simulink model "RoverA1Arch"  (R2026a)
settings: Solver=VariableStepAuto
model workspace (MAT data in the model file):
  averageLoad = Simulink.Parameter
  averageLoad.Value = 160
  averageLoad.Complexity = 'real'
  averageLoad.Dimensions = [1 1]
  averageLoad.DataType = 'double'
  averageLoad.DocUnits = 'W'
  bodyMass = Simulink.Parameter
  bodyMass.Value = 33.45
  bodyMass.Complexity = 'real'
  bodyMass.Dimensions = [1 1]
  bodyMass.DataType = 'double'
  bodyMass.DocUnits = 'kg'
  wheelSeparation = Simulink.Parameter
  wheelSeparation.Value = 0.62602
  wheelSeparation.Complexity = 'real'
  wheelSeparation.Dimensions = [1 1]
  wheelSeparation.DataType = 'double'
  wheelSeparation.DocUnits = 'm'
  wheelbase = Simulink.Parameter
  wheelbase.Value = 0.5084
  wheelbase.Complexity = 'real'
  wheelbase.Dimensions = [1 1]
  wheelbase.DataType = 'double'
  wheelbase.DocUnits = 'm'
settings Model: DataDictionary=RoverA1Interfaces.sldd  ParameterArgumentNames=bodyMass,wheelSeparation,wheelbase,averageLoad  Creator=potlo  LastModifiedBy=potlo

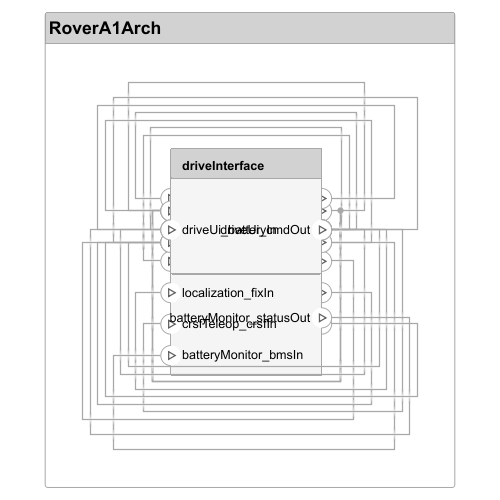
[thumbnail: Simulink's stored preview of the top-level diagram]
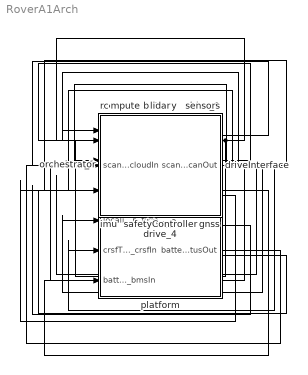
== system RoverA1Arch ==
  battery : Subsystem  mask{capacity=40, nominalVoltage=24}
      settings: PortSchema="{\"entries\":[{\"content\":{\"headerSize\":26,\"margin\":15,\"minimumSpacing\":25,\"sides\":[{\"content\":{},\"type\":\"ConnectorPlacement.EquallySpacedRectSide\",\"uuid\":\"200c6e72-70f4-4dab-9973-1633f40310af\"},{\"content\":{\"connectorIds\":[\"Out1\",\"Out2\"],\"side\":\"RIGHT\"},\"type\":\"ConnectorPlacement.EquallySpacedRectSide\",\"uuid\":\"bbe755dc-37e6-4ccf-babc-f69c624e3127\"},{\"content\":{\"side\":\"TOP\"},\"type\":\"ConnectorPlacement.EquallySpacedRectSide\",\"uuid\":\"af29013d-bc34-4ea7-a3b1-8488eaa61b9f\"}]},\"type\":\"ConnectorPlacement.EquallySpacedConnector\",\"uuid\":\"0c1b5d18-eb5c-4f03-ad77-d46c7555bc12\"}],\"packageUris\":[\"http://schema.mathworks.com/mf0/Connector/R2020b\"],\"version\":\"1.0\"}"
  compute : Subsystem
      settings: PortSchema="{\"entries\":[{\"content\":{\"headerSize\":26,\"margin\":15,\"minimumSpacing\":25,\"sides\":[{\"content\":{},\"type\":\"ConnectorPlacement.EquallySpacedRectSide\",\"uuid\":\"200c6e72-70f4-4dab-9973-1633f40310af\"},{\"content\":{\"connectorIds\":[\"Out1\",\"Out2\",\"Out3\",\"Out4\",\"Out5\"],\"side\":\"RIGHT\"},\"type\":\"ConnectorPlacement.EquallySpacedRectSide\",\"uuid\":\"bbe755dc-37e6-4ccf-babc-f69c624e3127\"},{\"content\":{\"side\":\"TOP\"},\"type\":\"ConnectorPlacement.EquallySpacedRectSide\",\"uuid\":\"af29013d-bc34-4ea7-a3b1-8488eaa61b9f\"}]},\"type\":\"ConnectorPlacement.EquallySpacedConnector\",\"uuid\":\"0c1b5d18-eb5c-4f03-ad77-d46c7555bc12\"}],\"packageUris\":[\"http://schema.mathworks.com/mf0/Connector/R2020b\"],\"version\":\"1.0\"}"
  driveInterface : Subsystem
      settings: PortSchema="{\"entries\":[{\"content\":{\"headerSize\":26,\"margin\":15,\"minimumSpacing\":25,\"sides\":[{\"content\":{\"connectorIds\":[\"In1\"]},\"type\":\"ConnectorPlacement.EquallySpacedRectSide\",\"uuid\":\"200c6e72-70f4-4dab-9973-1633f40310af\"},{\"content\":{\"connectorIds\":[\"Out1\"],\"side\":\"RIGHT\"},\"type\":\"ConnectorPlacement.EquallySpacedRectSide\",\"uuid\":\"bbe755dc-37e6-4ccf-babc-f69c624e3127\"},{\"content\":{\"side\":\"TOP\"},\"type\":\"ConnectorPlacement.EquallySpacedRectSide\",\"uuid\":\"af29013d-bc34-4ea7-a3b1-8488eaa61b9f\"}]},\"type\":\"ConnectorPlacement.EquallySpacedConnector\",\"uuid\":\"0c1b5d18-eb5c-4f03-ad77-d46c7555bc12\"}],\"packageUris\":[\"http://schema.mathworks.com/mf0/Connector/R2020b\"],\"version\":\"1.0\"}"
  drive_1 : Subsystem
      settings: PortSchema="{\"entries\":[{\"content\":{\"headerSize\":26,\"margin\":15,\"minimumSpacing\":25,\"sides\":[{\"content\":{\"connectorIds\":[\"In1\",\"In2\"]},\"type\":\"ConnectorPlacement.EquallySpacedRectSide\",\"uuid\":\"200c6e72-70f4-4dab-9973-1633f40310af\"},{\"content\":{\"side\":\"RIGHT\"},\"type\":\"ConnectorPlacement.EquallySpacedRectSide\",\"uuid\":\"bbe755dc-37e6-4ccf-babc-f69c624e3127\"},{\"content\":{\"side\":\"TOP\"},\"type\":\"ConnectorPlacement.EquallySpacedRectSide\",\"uuid\":\"af29013d-bc34-4ea7-a3b1-8488eaa61b9f\"}]},\"type\":\"ConnectorPlacement.EquallySpacedConnector\",\"uuid\":\"0c1b5d18-eb5c-4f03-ad77-d46c7555bc12\"}],\"packageUris\":[\"http://schema.mathworks.com/mf0/Connector/R2020b\"],\"version\":\"1.0\"}"
  drive_2 : Subsystem
      settings: PortSchema="{\"entries\":[{\"content\":{\"headerSize\":26,\"margin\":15,\"minimumSpacing\":25,\"sides\":[{\"content\":{\"connectorIds\":[\"In1\",\"In2\"]},\"type\":\"ConnectorPlacement.EquallySpacedRectSide\",\"uuid\":\"200c6e72-70f4-4dab-9973-1633f40310af\"},{\"content\":{\"side\":\"RIGHT\"},\"type\":\"ConnectorPlacement.EquallySpacedRectSide\",\"uuid\":\"bbe755dc-37e6-4ccf-babc-f69c624e3127\"},{\"content\":{\"side\":\"TOP\"},\"type\":\"ConnectorPlacement.EquallySpacedRectSide\",\"uuid\":\"af29013d-bc34-4ea7-a3b1-8488eaa61b9f\"}]},\"type\":\"ConnectorPlacement.EquallySpacedConnector\",\"uuid\":\"0c1b5d18-eb5c-4f03-ad77-d46c7555bc12\"}],\"packageUris\":[\"http://schema.mathworks.com/mf0/Connector/R2020b\"],\"version\":\"1.0\"}"
  drive_3 : Subsystem
      settings: PortSchema="{\"entries\":[{\"content\":{\"headerSize\":26,\"margin\":15,\"minimumSpacing\":25,\"sides\":[{\"content\":{\"connectorIds\":[\"In1\",\"In2\"]},\"type\":\"ConnectorPlacement.EquallySpacedRectSide\",\"uuid\":\"200c6e72-70f4-4dab-9973-1633f40310af\"},{\"content\":{\"side\":\"RIGHT\"},\"type\":\"ConnectorPlacement.EquallySpacedRectSide\",\"uuid\":\"bbe755dc-37e6-4ccf-babc-f69c624e3127\"},{\"content\":{\"side\":\"TOP\"},\"type\":\"ConnectorPlacement.EquallySpacedRectSide\",\"uuid\":\"af29013d-bc34-4ea7-a3b1-8488eaa61b9f\"}]},\"type\":\"ConnectorPlacement.EquallySpacedConnector\",\"uuid\":\"0c1b5d18-eb5c-4f03-ad77-d46c7555bc12\"}],\"packageUris\":[\"http://schema.mathworks.com/mf0/Connector/R2020b\"],\"version\":\"1.0\"}"
  drive_4 : Subsystem
      settings: PortSchema="{\"entries\":[{\"content\":{\"headerSize\":26,\"margin\":15,\"minimumSpacing\":25,\"sides\":[{\"content\":{\"connectorIds\":[\"In1\",\"In2\"]},\"type\":\"ConnectorPlacement.EquallySpacedRectSide\",\"uuid\":\"200c6e72-70f4-4dab-9973-1633f40310af\"},{\"content\":{\"side\":\"RIGHT\"},\"type\":\"ConnectorPlacement.EquallySpacedRectSide\",\"uuid\":\"bbe755dc-37e6-4ccf-babc-f69c624e3127\"},{\"content\":{\"side\":\"TOP\"},\"type\":\"ConnectorPlacement.EquallySpacedRectSide\",\"uuid\":\"af29013d-bc34-4ea7-a3b1-8488eaa61b9f\"}]},\"type\":\"ConnectorPlacement.EquallySpacedConnector\",\"uuid\":\"0c1b5d18-eb5c-4f03-ad77-d46c7555bc12\"}],\"packageUris\":[\"http://schema.mathworks.com/mf0/Connector/R2020b\"],\"version\":\"1.0\"}"
  gnss : Subsystem  mask{fixRate=1}
      settings: PortSchema="{\"entries\":[{\"content\":{\"headerSize\":26,\"margin\":15,\"minimumSpacing\":25,\"sides\":[{\"content\":{},\"type\":\"ConnectorPlacement.EquallySpacedRectSide\",\"uuid\":\"200c6e72-70f4-4dab-9973-1633f40310af\"},{\"content\":{\"connectorIds\":[\"Out1\"],\"side\":\"RIGHT\"},\"type\":\"ConnectorPlacement.EquallySpacedRectSide\",\"uuid\":\"bbe755dc-37e6-4ccf-babc-f69c624e3127\"},{\"content\":{\"side\":\"TOP\"},\"type\":\"ConnectorPlacement.EquallySpacedRectSide\",\"uuid\":\"af29013d-bc34-4ea7-a3b1-8488eaa61b9f\"}]},\"type\":\"ConnectorPlacement.EquallySpacedConnector\",\"uuid\":\"0c1b5d18-eb5c-4f03-ad77-d46c7555bc12\"}],\"packageUris\":[\"http://schema.mathworks.com/mf0/Connector/R2020b\"],\"version\":\"1.0\"}"
  imu : Subsystem
      settings: PortSchema="{\"entries\":[{\"content\":{\"headerSize\":26,\"margin\":15,\"minimumSpacing\":25,\"sides\":[{\"content\":{},\"type\":\"ConnectorPlacement.EquallySpacedRectSide\",\"uuid\":\"200c6e72-70f4-4dab-9973-1633f40310af\"},{\"content\":{\"connectorIds\":[\"Out1\"],\"side\":\"RIGHT\"},\"type\":\"ConnectorPlacement.EquallySpacedRectSide\",\"uuid\":\"bbe755dc-37e6-4ccf-babc-f69c624e3127\"},{\"content\":{\"side\":\"TOP\"},\"type\":\"ConnectorPlacement.EquallySpacedRectSide\",\"uuid\":\"af29013d-bc34-4ea7-a3b1-8488eaa61b9f\"}]},\"type\":\"ConnectorPlacement.EquallySpacedConnector\",\"uuid\":\"0c1b5d18-eb5c-4f03-ad77-d46c7555bc12\"}],\"packageUris\":[\"http://schema.mathworks.com/mf0/Connector/R2020b\"],\"version\":\"1.0\"}"
  lidar : Subsystem  mask{scanRate=10}
      settings: PortSchema="{\"entries\":[{\"content\":{\"headerSize\":26,\"margin\":15,\"minimumSpacing\":25,\"sides\":[{\"content\":{},\"type\":\"ConnectorPlacement.EquallySpacedRectSide\",\"uuid\":\"200c6e72-70f4-4dab-9973-1633f40310af\"},{\"content\":{\"connectorIds\":[\"Out1\"],\"side\":\"RIGHT\"},\"type\":\"ConnectorPlacement.EquallySpacedRectSide\",\"uuid\":\"bbe755dc-37e6-4ccf-babc-f69c624e3127\"},{\"content\":{\"side\":\"TOP\"},\"type\":\"ConnectorPlacement.EquallySpacedRectSide\",\"uuid\":\"af29013d-bc34-4ea7-a3b1-8488eaa61b9f\"}]},\"type\":\"ConnectorPlacement.EquallySpacedConnector\",\"uuid\":\"0c1b5d18-eb5c-4f03-ad77-d46c7555bc12\"}],\"packageUris\":[\"http://schema.mathworks.com/mf0/Connector/R2020b\"],\"version\":\"1.0\"}"
  orchestrator : Subsystem
      settings: PortSchema="{\"entries\":[{\"content\":{\"headerSize\":26,\"margin\":15,\"minimumSpacing\":25,\"sides\":[{\"content\":{\"connectorIds\":[\"In1\",\"In2\"]},\"type\":\"ConnectorPlacement.EquallySpacedRectSide\",\"uuid\":\"200c6e72-70f4-4dab-9973-1633f40310af\"},{\"content\":{\"connectorIds\":[\"Out1\"],\"side\":\"RIGHT\"},\"type\":\"ConnectorPlacement.EquallySpacedRectSide\",\"uuid\":\"bbe755dc-37e6-4ccf-babc-f69c624e3127\"},{\"content\":{\"side\":\"TOP\"},\"type\":\"ConnectorPlacement.EquallySpacedRectSide\",\"uuid\":\"af29013d-bc34-4ea7-a3b1-8488eaa61b9f\"}]},\"type\":\"ConnectorPlacement.EquallySpacedConnector\",\"uuid\":\"0c1b5d18-eb5c-4f03-ad77-d46c7555bc12\"}],\"packageUris\":[\"http://schema.mathworks.com/mf0/Connector/R2020b\"],\"version\":\"1.0\"}"
  platform : Subsystem
      settings: PortSchema="{\"entries\":[{\"content\":{\"headerSize\":26,\"margin\":15,\"minimumSpacing\":25,\"sides\":[{\"content\":{\"connectorIds\":[\"In1\",\"In2\",\"In3\",\"In4\",\"In5\",\"In6\"]},\"type\":\"ConnectorPlacement.EquallySpacedRectSide\",\"uuid\":\"200c6e72-70f4-4dab-9973-1633f40310af\"},{\"content\":{\"connectorIds\":[\"Out1\",\"Out2\"],\"side\":\"RIGHT\"},\"type\":\"ConnectorPlacement.EquallySpacedRectSide\",\"uuid\":\"bbe755dc-37e6-4ccf-babc-f69c624e3127\"},{\"content\":{\"side\":\"TOP\"},\"type\":\"ConnectorPlacement.EquallySpacedRectSide\",\"uuid\":\"af29013d-bc34-4ea7-a3b1-8488eaa61b9f\"}]},\"type\":\"ConnectorPlacement.EquallySpacedConnector\",\"uuid\":\"0c1b5d18-eb5c-4f03-ad77-d46c7555bc12\"}],\"packageUris\":[\"http://schema.mathworks.com/mf0/Connector/R2020b\"],\"version\":\"1.0\"}"
  rc : Subsystem
      settings: PortSchema="{\"entries\":[{\"content\":{\"headerSize\":26,\"margin\":15,\"minimumSpacing\":25,\"sides\":[{\"content\":{},\"type\":\"ConnectorPlacement.EquallySpacedRectSide\",\"uuid\":\"200c6e72-70f4-4dab-9973-1633f40310af\"},{\"content\":{\"connectorIds\":[\"Out1\"],\"side\":\"RIGHT\"},\"type\":\"ConnectorPlacement.EquallySpacedRectSide\",\"uuid\":\"bbe755dc-37e6-4ccf-babc-f69c624e3127\"},{\"content\":{\"side\":\"TOP\"},\"type\":\"ConnectorPlacement.EquallySpacedRectSide\",\"uuid\":\"af29013d-bc34-4ea7-a3b1-8488eaa61b9f\"}]},\"type\":\"ConnectorPlacement.EquallySpacedConnector\",\"uuid\":\"0c1b5d18-eb5c-4f03-ad77-d46c7555bc12\"}],\"packageUris\":[\"http://schema.mathworks.com/mf0/Connector/R2020b\"],\"version\":\"1.0\"}"
  safetyController : Subsystem  mask{watchdogPeriod=0.2}
      settings: PortSchema="{\"entries\":[{\"content\":{\"headerSize\":26,\"margin\":15,\"minimumSpacing\":25,\"sides\":[{\"content\":{\"connectorIds\":[\"In1\"]},\"type\":\"ConnectorPlacement.EquallySpacedRectSide\",\"uuid\":\"200c6e72-70f4-4dab-9973-1633f40310af\"},{\"content\":{\"side\":\"RIGHT\"},\"type\":\"ConnectorPlacement.EquallySpacedRectSide\",\"uuid\":\"bbe755dc-37e6-4ccf-babc-f69c624e3127\"},{\"content\":{\"side\":\"TOP\"},\"type\":\"ConnectorPlacement.EquallySpacedRectSide\",\"uuid\":\"af29013d-bc34-4ea7-a3b1-8488eaa61b9f\"}]},\"type\":\"ConnectorPlacement.EquallySpacedConnector\",\"uuid\":\"0c1b5d18-eb5c-4f03-ad77-d46c7555bc12\"}],\"packageUris\":[\"http://schema.mathworks.com/mf0/Connector/R2020b\"],\"version\":\"1.0\"}"
  sensors : Subsystem
      settings: PortSchema="{\"entries\":[{\"content\":{\"headerSize\":26,\"margin\":15,\"minimumSpacing\":25,\"sides\":[{\"content\":{\"connectorIds\":[\"In1\"]},\"type\":\"ConnectorPlacement.EquallySpacedRectSide\",\"uuid\":\"200c6e72-70f4-4dab-9973-1633f40310af\"},{\"content\":{\"connectorIds\":[\"Out1\"],\"side\":\"RIGHT\"},\"type\":\"ConnectorPlacement.EquallySpacedRectSide\",\"uuid\":\"bbe755dc-37e6-4ccf-babc-f69c624e3127\"},{\"content\":{\"side\":\"TOP\"},\"type\":\"ConnectorPlacement.EquallySpacedRectSide\",\"uuid\":\"af29013d-bc34-4ea7-a3b1-8488eaa61b9f\"}]},\"type\":\"ConnectorPlacement.EquallySpacedConnector\",\"uuid\":\"0c1b5d18-eb5c-4f03-ad77-d46c7555bc12\"}],\"packageUris\":[\"http://schema.mathworks.com/mf0/Connector/R2020b\"],\"version\":\"1.0\"}"
  wires:
  driveInterface/1(driveUi_cmdOut) -> platform/1(twistMux_webIn)
  orchestrator/1(navigation_cmdOut) -> platform/2(twistMux_navIn)
  imu/1(imuOut) -> platform/3(localization_imuIn)
  gnss/1(fixOut) -> platform/4(localization_fixIn)
  platform/1(localization_odomOut) -> orchestrator/1(navigation_odomIn)
  lidar/1(cloudOut) -> sensors/1(scanProjection_cloudIn)
  sensors/1(scanProjection_scanOut) -> orchestrator/2(navigation_scanIn)
  battery/1(powerOut) -> drive_1/1(controller_powerIn), drive_2/1(controller_powerIn), drive_3/1(controller_powerIn), drive_4/1(controller_powerIn)
  compute/2(wheelCmdOut_1) -> drive_1/2(controller_wheelCmdIn)
  compute/3(wheelCmdOut_2) -> drive_2/2(controller_wheelCmdIn)
  compute/4(wheelCmdOut_3) -> drive_3/2(controller_wheelCmdIn)
  compute/5(wheelCmdOut_4) -> drive_4/2(controller_wheelCmdIn)
  rc/1(crsfOut) -> platform/5(crsfTeleop_crsfIn)
  battery/2(statusOut) -> platform/6(batteryMonitor_bmsIn)
  platform/2(batteryMonitor_statusOut) -> driveInterface/1(driveUi_batteryIn)
  compute/1(modbus) -> safetyController/1(modbus)

== system RoverA1Arch/battery ==
  Bus Element Out1 : Outport  PortName=powerOut
  Bus Element Out2 : Outport  Port=2  PortName=statusOut

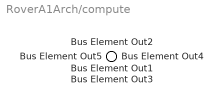
== system RoverA1Arch/compute ==
  Bus Element Out1 : Outport  PortName=modbus
  Bus Element Out2 : Outport  Port=2  PortName=wheelCmdOut_1
  Bus Element Out3 : Outport  Port=3  PortName=wheelCmdOut_2
  Bus Element Out4 : Outport  Port=4  PortName=wheelCmdOut_3
  Bus Element Out5 : Outport  Port=5  PortName=wheelCmdOut_4

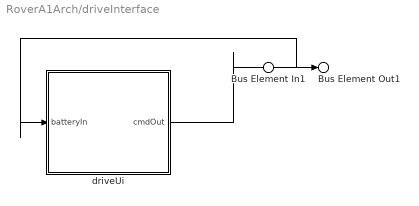
== system RoverA1Arch/driveInterface ==
  Bus Element In1 : Inport  PortName=driveUi_batteryIn
  driveUi : Subsystem
      settings: PortSchema="{\"entries\":[{\"content\":{\"headerSize\":26,\"margin\":15,\"minimumSpacing\":25,\"sides\":[{\"content\":{\"connectorIds\":[\"In1\"]},\"type\":\"ConnectorPlacement.EquallySpacedRectSide\",\"uuid\":\"200c6e72-70f4-4dab-9973-1633f40310af\"},{\"content\":{\"connectorIds\":[\"Out1\"],\"side\":\"RIGHT\"},\"type\":\"ConnectorPlacement.EquallySpacedRectSide\",\"uuid\":\"bbe755dc-37e6-4ccf-babc-f69c624e3127\"},{\"content\":{\"side\":\"TOP\"},\"type\":\"ConnectorPlacement.EquallySpacedRectSide\",\"uuid\":\"af29013d-bc34-4ea7-a3b1-8488eaa61b9f\"}]},\"type\":\"ConnectorPlacement.EquallySpacedConnector\",\"uuid\":\"0c1b5d18-eb5c-4f03-ad77-d46c7555bc12\"}],\"packageUris\":[\"http://schema.mathworks.com/mf0/Connector/R2020b\"],\"version\":\"1.0\"}"
  Bus Element Out1 : Outport  PortName=driveUi_cmdOut
  wires:
  driveUi/1(cmdOut) -> Bus Element Out1/1
  Bus Element In1/1 -> driveUi/1(batteryIn)

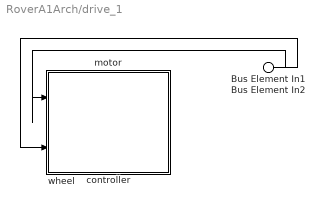
== system RoverA1Arch/drive_1 ==
  Bus Element In1 : Inport  PortName=controller_powerIn
  Bus Element In2 : Inport  Port=2  PortName=controller_wheelCmdIn
  controller : Subsystem
      settings: PortSchema="{\"entries\":[{\"content\":{\"headerSize\":26,\"margin\":15,\"minimumSpacing\":25,\"sides\":[{\"content\":{\"connectorIds\":[\"In1\",\"In2\"]},\"type\":\"ConnectorPlacement.EquallySpacedRectSide\",\"uuid\":\"200c6e72-70f4-4dab-9973-1633f40310af\"},{\"content\":{\"side\":\"RIGHT\"},\"type\":\"ConnectorPlacement.EquallySpacedRectSide\",\"uuid\":\"bbe755dc-37e6-4ccf-babc-f69c624e3127\"},{\"content\":{\"side\":\"TOP\"},\"type\":\"ConnectorPlacement.EquallySpacedRectSide\",\"uuid\":\"af29013d-bc34-4ea7-a3b1-8488eaa61b9f\"}]},\"type\":\"ConnectorPlacement.EquallySpacedConnector\",\"uuid\":\"0c1b5d18-eb5c-4f03-ad77-d46c7555bc12\"}],\"packageUris\":[\"http://schema.mathworks.com/mf0/Connector/R2020b\"],\"version\":\"1.0\"}"
  motor : Subsystem  mask{noLoadSpeed=293.2, gearRatio=23.3, gearboxEfficiency=0.70, currentLimit=15, jointVelocityLimit=10.958}
      settings: PortSchema="{\"entries\":[{\"content\":{\"headerSize\":26,\"margin\":15,\"minimumSpacing\":25,\"sides\":[{\"content\":{},\"type\":\"ConnectorPlacement.EquallySpacedRectSide\",\"uuid\":\"200c6e72-70f4-4dab-9973-1633f40310af\"},{\"content\":{\"side\":\"RIGHT\"},\"type\":\"ConnectorPlacement.EquallySpacedRectSide\",\"uuid\":\"bbe755dc-37e6-4ccf-babc-f69c624e3127\"},{\"content\":{\"side\":\"TOP\"},\"type\":\"ConnectorPlacement.EquallySpacedRectSide\",\"uuid\":\"af29013d-bc34-4ea7-a3b1-8488eaa61b9f\"}]},\"type\":\"ConnectorPlacement.EquallySpacedConnector\",\"uuid\":\"0c1b5d18-eb5c-4f03-ad77-d46c7555bc12\"}],\"packageUris\":[\"http://schema.mathworks.com/mf0/Connector/R2020b\"],\"version\":\"1.0\"}"
  wheel : Subsystem  mask{radius=0.1651, width=0.108, mass=2.5}
      settings: PortSchema="{\"entries\":[{\"content\":{\"headerSize\":26,\"margin\":15,\"minimumSpacing\":25,\"sides\":[{\"content\":{},\"type\":\"ConnectorPlacement.EquallySpacedRectSide\",\"uuid\":\"200c6e72-70f4-4dab-9973-1633f40310af\"},{\"content\":{\"side\":\"RIGHT\"},\"type\":\"ConnectorPlacement.EquallySpacedRectSide\",\"uuid\":\"bbe755dc-37e6-4ccf-babc-f69c624e3127\"},{\"content\":{\"side\":\"TOP\"},\"type\":\"ConnectorPlacement.EquallySpacedRectSide\",\"uuid\":\"af29013d-bc34-4ea7-a3b1-8488eaa61b9f\"}]},\"type\":\"ConnectorPlacement.EquallySpacedConnector\",\"uuid\":\"0c1b5d18-eb5c-4f03-ad77-d46c7555bc12\"}],\"packageUris\":[\"http://schema.mathworks.com/mf0/Connector/R2020b\"],\"version\":\"1.0\"}"
  wires:
  Bus Element In1/1 -> controller/2(powerIn)
  Bus Element In2/1 -> controller/1(wheelCmdIn)

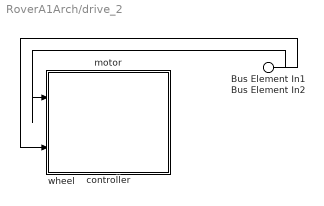
== system RoverA1Arch/drive_2 ==
  Bus Element In1 : Inport  PortName=controller_powerIn
  Bus Element In2 : Inport  Port=2  PortName=controller_wheelCmdIn
  controller : Subsystem
      settings: PortSchema="{\"entries\":[{\"content\":{\"headerSize\":26,\"margin\":15,\"minimumSpacing\":25,\"sides\":[{\"content\":{\"connectorIds\":[\"In1\",\"In2\"]},\"type\":\"ConnectorPlacement.EquallySpacedRectSide\",\"uuid\":\"200c6e72-70f4-4dab-9973-1633f40310af\"},{\"content\":{\"side\":\"RIGHT\"},\"type\":\"ConnectorPlacement.EquallySpacedRectSide\",\"uuid\":\"bbe755dc-37e6-4ccf-babc-f69c624e3127\"},{\"content\":{\"side\":\"TOP\"},\"type\":\"ConnectorPlacement.EquallySpacedRectSide\",\"uuid\":\"af29013d-bc34-4ea7-a3b1-8488eaa61b9f\"}]},\"type\":\"ConnectorPlacement.EquallySpacedConnector\",\"uuid\":\"0c1b5d18-eb5c-4f03-ad77-d46c7555bc12\"}],\"packageUris\":[\"http://schema.mathworks.com/mf0/Connector/R2020b\"],\"version\":\"1.0\"}"
  motor : Subsystem  mask{noLoadSpeed=293.2, gearRatio=23.3, gearboxEfficiency=0.70, currentLimit=15, jointVelocityLimit=10.958}
      settings: PortSchema="{\"entries\":[{\"content\":{\"headerSize\":26,\"margin\":15,\"minimumSpacing\":25,\"sides\":[{\"content\":{},\"type\":\"ConnectorPlacement.EquallySpacedRectSide\",\"uuid\":\"200c6e72-70f4-4dab-9973-1633f40310af\"},{\"content\":{\"side\":\"RIGHT\"},\"type\":\"ConnectorPlacement.EquallySpacedRectSide\",\"uuid\":\"bbe755dc-37e6-4ccf-babc-f69c624e3127\"},{\"content\":{\"side\":\"TOP\"},\"type\":\"ConnectorPlacement.EquallySpacedRectSide\",\"uuid\":\"af29013d-bc34-4ea7-a3b1-8488eaa61b9f\"}]},\"type\":\"ConnectorPlacement.EquallySpacedConnector\",\"uuid\":\"0c1b5d18-eb5c-4f03-ad77-d46c7555bc12\"}],\"packageUris\":[\"http://schema.mathworks.com/mf0/Connector/R2020b\"],\"version\":\"1.0\"}"
  wheel : Subsystem  mask{radius=0.1651, width=0.108, mass=2.5}
      settings: PortSchema="{\"entries\":[{\"content\":{\"headerSize\":26,\"margin\":15,\"minimumSpacing\":25,\"sides\":[{\"content\":{},\"type\":\"ConnectorPlacement.EquallySpacedRectSide\",\"uuid\":\"200c6e72-70f4-4dab-9973-1633f40310af\"},{\"content\":{\"side\":\"RIGHT\"},\"type\":\"ConnectorPlacement.EquallySpacedRectSide\",\"uuid\":\"bbe755dc-37e6-4ccf-babc-f69c624e3127\"},{\"content\":{\"side\":\"TOP\"},\"type\":\"ConnectorPlacement.EquallySpacedRectSide\",\"uuid\":\"af29013d-bc34-4ea7-a3b1-8488eaa61b9f\"}]},\"type\":\"ConnectorPlacement.EquallySpacedConnector\",\"uuid\":\"0c1b5d18-eb5c-4f03-ad77-d46c7555bc12\"}],\"packageUris\":[\"http://schema.mathworks.com/mf0/Connector/R2020b\"],\"version\":\"1.0\"}"
  wires:
  Bus Element In1/1 -> controller/2(powerIn)
  Bus Element In2/1 -> controller/1(wheelCmdIn)

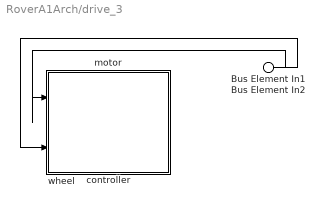
== system RoverA1Arch/drive_3 ==
  Bus Element In1 : Inport  PortName=controller_powerIn
  Bus Element In2 : Inport  Port=2  PortName=controller_wheelCmdIn
  controller : Subsystem
      settings: PortSchema="{\"entries\":[{\"content\":{\"headerSize\":26,\"margin\":15,\"minimumSpacing\":25,\"sides\":[{\"content\":{\"connectorIds\":[\"In1\",\"In2\"]},\"type\":\"ConnectorPlacement.EquallySpacedRectSide\",\"uuid\":\"200c6e72-70f4-4dab-9973-1633f40310af\"},{\"content\":{\"side\":\"RIGHT\"},\"type\":\"ConnectorPlacement.EquallySpacedRectSide\",\"uuid\":\"bbe755dc-37e6-4ccf-babc-f69c624e3127\"},{\"content\":{\"side\":\"TOP\"},\"type\":\"ConnectorPlacement.EquallySpacedRectSide\",\"uuid\":\"af29013d-bc34-4ea7-a3b1-8488eaa61b9f\"}]},\"type\":\"ConnectorPlacement.EquallySpacedConnector\",\"uuid\":\"0c1b5d18-eb5c-4f03-ad77-d46c7555bc12\"}],\"packageUris\":[\"http://schema.mathworks.com/mf0/Connector/R2020b\"],\"version\":\"1.0\"}"
  motor : Subsystem  mask{noLoadSpeed=293.2, gearRatio=23.3, gearboxEfficiency=0.70, currentLimit=15, jointVelocityLimit=10.958}
      settings: PortSchema="{\"entries\":[{\"content\":{\"headerSize\":26,\"margin\":15,\"minimumSpacing\":25,\"sides\":[{\"content\":{},\"type\":\"ConnectorPlacement.EquallySpacedRectSide\",\"uuid\":\"200c6e72-70f4-4dab-9973-1633f40310af\"},{\"content\":{\"side\":\"RIGHT\"},\"type\":\"ConnectorPlacement.EquallySpacedRectSide\",\"uuid\":\"bbe755dc-37e6-4ccf-babc-f69c624e3127\"},{\"content\":{\"side\":\"TOP\"},\"type\":\"ConnectorPlacement.EquallySpacedRectSide\",\"uuid\":\"af29013d-bc34-4ea7-a3b1-8488eaa61b9f\"}]},\"type\":\"ConnectorPlacement.EquallySpacedConnector\",\"uuid\":\"0c1b5d18-eb5c-4f03-ad77-d46c7555bc12\"}],\"packageUris\":[\"http://schema.mathworks.com/mf0/Connector/R2020b\"],\"version\":\"1.0\"}"
  wheel : Subsystem  mask{radius=0.1651, width=0.108, mass=2.5}
      settings: PortSchema="{\"entries\":[{\"content\":{\"headerSize\":26,\"margin\":15,\"minimumSpacing\":25,\"sides\":[{\"content\":{},\"type\":\"ConnectorPlacement.EquallySpacedRectSide\",\"uuid\":\"200c6e72-70f4-4dab-9973-1633f40310af\"},{\"content\":{\"side\":\"RIGHT\"},\"type\":\"ConnectorPlacement.EquallySpacedRectSide\",\"uuid\":\"bbe755dc-37e6-4ccf-babc-f69c624e3127\"},{\"content\":{\"side\":\"TOP\"},\"type\":\"ConnectorPlacement.EquallySpacedRectSide\",\"uuid\":\"af29013d-bc34-4ea7-a3b1-8488eaa61b9f\"}]},\"type\":\"ConnectorPlacement.EquallySpacedConnector\",\"uuid\":\"0c1b5d18-eb5c-4f03-ad77-d46c7555bc12\"}],\"packageUris\":[\"http://schema.mathworks.com/mf0/Connector/R2020b\"],\"version\":\"1.0\"}"
  wires:
  Bus Element In1/1 -> controller/2(powerIn)
  Bus Element In2/1 -> controller/1(wheelCmdIn)

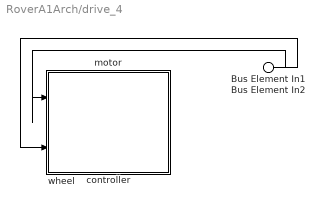
== system RoverA1Arch/drive_4 ==
  Bus Element In1 : Inport  PortName=controller_powerIn
  Bus Element In2 : Inport  Port=2  PortName=controller_wheelCmdIn
  controller : Subsystem
      settings: PortSchema="{\"entries\":[{\"content\":{\"headerSize\":26,\"margin\":15,\"minimumSpacing\":25,\"sides\":[{\"content\":{\"connectorIds\":[\"In1\",\"In2\"]},\"type\":\"ConnectorPlacement.EquallySpacedRectSide\",\"uuid\":\"200c6e72-70f4-4dab-9973-1633f40310af\"},{\"content\":{\"side\":\"RIGHT\"},\"type\":\"ConnectorPlacement.EquallySpacedRectSide\",\"uuid\":\"bbe755dc-37e6-4ccf-babc-f69c624e3127\"},{\"content\":{\"side\":\"TOP\"},\"type\":\"ConnectorPlacement.EquallySpacedRectSide\",\"uuid\":\"af29013d-bc34-4ea7-a3b1-8488eaa61b9f\"}]},\"type\":\"ConnectorPlacement.EquallySpacedConnector\",\"uuid\":\"0c1b5d18-eb5c-4f03-ad77-d46c7555bc12\"}],\"packageUris\":[\"http://schema.mathworks.com/mf0/Connector/R2020b\"],\"version\":\"1.0\"}"
  motor : Subsystem  mask{noLoadSpeed=293.2, gearRatio=23.3, gearboxEfficiency=0.70, currentLimit=15, jointVelocityLimit=10.958}
      settings: PortSchema="{\"entries\":[{\"content\":{\"headerSize\":26,\"margin\":15,\"minimumSpacing\":25,\"sides\":[{\"content\":{},\"type\":\"ConnectorPlacement.EquallySpacedRectSide\",\"uuid\":\"200c6e72-70f4-4dab-9973-1633f40310af\"},{\"content\":{\"side\":\"RIGHT\"},\"type\":\"ConnectorPlacement.EquallySpacedRectSide\",\"uuid\":\"bbe755dc-37e6-4ccf-babc-f69c624e3127\"},{\"content\":{\"side\":\"TOP\"},\"type\":\"ConnectorPlacement.EquallySpacedRectSide\",\"uuid\":\"af29013d-bc34-4ea7-a3b1-8488eaa61b9f\"}]},\"type\":\"ConnectorPlacement.EquallySpacedConnector\",\"uuid\":\"0c1b5d18-eb5c-4f03-ad77-d46c7555bc12\"}],\"packageUris\":[\"http://schema.mathworks.com/mf0/Connector/R2020b\"],\"version\":\"1.0\"}"
  wheel : Subsystem  mask{radius=0.1651, width=0.108, mass=2.5}
      settings: PortSchema="{\"entries\":[{\"content\":{\"headerSize\":26,\"margin\":15,\"minimumSpacing\":25,\"sides\":[{\"content\":{},\"type\":\"ConnectorPlacement.EquallySpacedRectSide\",\"uuid\":\"200c6e72-70f4-4dab-9973-1633f40310af\"},{\"content\":{\"side\":\"RIGHT\"},\"type\":\"ConnectorPlacement.EquallySpacedRectSide\",\"uuid\":\"bbe755dc-37e6-4ccf-babc-f69c624e3127\"},{\"content\":{\"side\":\"TOP\"},\"type\":\"ConnectorPlacement.EquallySpacedRectSide\",\"uuid\":\"af29013d-bc34-4ea7-a3b1-8488eaa61b9f\"}]},\"type\":\"ConnectorPlacement.EquallySpacedConnector\",\"uuid\":\"0c1b5d18-eb5c-4f03-ad77-d46c7555bc12\"}],\"packageUris\":[\"http://schema.mathworks.com/mf0/Connector/R2020b\"],\"version\":\"1.0\"}"
  wires:
  Bus Element In1/1 -> controller/2(powerIn)
  Bus Element In2/1 -> controller/1(wheelCmdIn)

== system RoverA1Arch/gnss ==
  Bus Element Out1 : Outport  PortName=fixOut

== system RoverA1Arch/imu ==
  Bus Element Out1 : Outport  PortName=imuOut

== system RoverA1Arch/lidar ==
  Bus Element Out1 : Outport  PortName=cloudOut

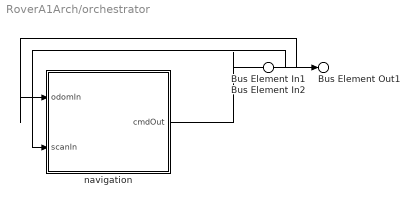
== system RoverA1Arch/orchestrator ==
  Bus Element In1 : Inport  PortName=navigation_odomIn
  Bus Element In2 : Inport  Port=2  PortName=navigation_scanIn
  navigation : Subsystem  mask{maxForwardSpeed=0.8, maxReverseSpeed=0.5, footprintRadius=0.693}
      settings: PortSchema="{\"entries\":[{\"content\":{\"headerSize\":26,\"margin\":15,\"minimumSpacing\":25,\"sides\":[{\"content\":{\"connectorIds\":[\"In1\",\"In2\"]},\"type\":\"ConnectorPlacement.EquallySpacedRectSide\",\"uuid\":\"200c6e72-70f4-4dab-9973-1633f40310af\"},{\"content\":{\"connectorIds\":[\"Out1\"],\"side\":\"RIGHT\"},\"type\":\"ConnectorPlacement.EquallySpacedRectSide\",\"uuid\":\"bbe755dc-37e6-4ccf-babc-f69c624e3127\"},{\"content\":{\"side\":\"TOP\"},\"type\":\"ConnectorPlacement.EquallySpacedRectSide\",\"uuid\":\"af29013d-bc34-4ea7-a3b1-8488eaa61b9f\"}]},\"type\":\"ConnectorPlacement.EquallySpacedConnector\",\"uuid\":\"0c1b5d18-eb5c-4f03-ad77-d46c7555bc12\"}],\"packageUris\":[\"http://schema.mathworks.com/mf0/Connector/R2020b\"],\"version\":\"1.0\"}"
  Bus Element Out1 : Outport  PortName=navigation_cmdOut
  wires:
  navigation/1(cmdOut) -> Bus Element Out1/1
  Bus Element In1/1 -> navigation/1(odomIn)
  Bus Element In2/1 -> navigation/2(scanIn)

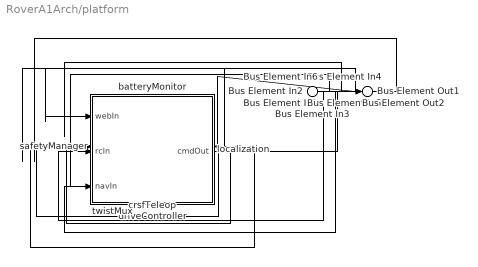
== system RoverA1Arch/platform ==
  Bus Element In1 : Inport  PortName=twistMux_webIn
  Bus Element In2 : Inport  Port=2  PortName=twistMux_navIn
  Bus Element In3 : Inport  Port=3  PortName=localization_imuIn
  Bus Element In4 : Inport  Port=4  PortName=localization_fixIn
  Bus Element In5 : Inport  Port=5  PortName=crsfTeleop_crsfIn
  Bus Element In6 : Inport  Port=6  PortName=batteryMonitor_bmsIn
  batteryMonitor : Subsystem
      settings: PortSchema="{\"entries\":[{\"content\":{\"headerSize\":26,\"margin\":15,\"minimumSpacing\":25,\"sides\":[{\"content\":{\"connectorIds\":[\"In1\"]},\"type\":\"ConnectorPlacement.EquallySpacedRectSide\",\"uuid\":\"200c6e72-70f4-4dab-9973-1633f40310af\"},{\"content\":{\"connectorIds\":[\"Out1\"],\"side\":\"RIGHT\"},\"type\":\"ConnectorPlacement.EquallySpacedRectSide\",\"uuid\":\"bbe755dc-37e6-4ccf-babc-f69c624e3127\"},{\"content\":{\"side\":\"TOP\"},\"type\":\"ConnectorPlacement.EquallySpacedRectSide\",\"uuid\":\"af29013d-bc34-4ea7-a3b1-8488eaa61b9f\"}]},\"type\":\"ConnectorPlacement.EquallySpacedConnector\",\"uuid\":\"0c1b5d18-eb5c-4f03-ad77-d46c7555bc12\"}],\"packageUris\":[\"http://schema.mathworks.com/mf0/Connector/R2020b\"],\"version\":\"1.0\"}"
  crsfTeleop : Subsystem
      settings: PortSchema="{\"entries\":[{\"content\":{\"headerSize\":26,\"margin\":15,\"minimumSpacing\":25,\"sides\":[{\"content\":{\"connectorIds\":[\"In1\"]},\"type\":\"ConnectorPlacement.EquallySpacedRectSide\",\"uuid\":\"200c6e72-70f4-4dab-9973-1633f40310af\"},{\"content\":{\"connectorIds\":[\"Out1\"],\"side\":\"RIGHT\"},\"type\":\"ConnectorPlacement.EquallySpacedRectSide\",\"uuid\":\"bbe755dc-37e6-4ccf-babc-f69c624e3127\"},{\"content\":{\"side\":\"TOP\"},\"type\":\"ConnectorPlacement.EquallySpacedRectSide\",\"uuid\":\"af29013d-bc34-4ea7-a3b1-8488eaa61b9f\"}]},\"type\":\"ConnectorPlacement.EquallySpacedConnector\",\"uuid\":\"0c1b5d18-eb5c-4f03-ad77-d46c7555bc12\"}],\"packageUris\":[\"http://schema.mathworks.com/mf0/Connector/R2020b\"],\"version\":\"1.0\"}"
  driveController : Subsystem  mask{updateRate=100, maxLinearSpeed=1.2, maxLinearAccel=2.7, maxAngularSpeed=1.0, cmdTimeout=0.5}
      settings: PortSchema="{\"entries\":[{\"content\":{\"headerSize\":26,\"margin\":15,\"minimumSpacing\":25,\"sides\":[{\"content\":{\"connectorIds\":[\"In1\"]},\"type\":\"ConnectorPlacement.EquallySpacedRectSide\",\"uuid\":\"200c6e72-70f4-4dab-9973-1633f40310af\"},{\"content\":{\"connectorIds\":[\"Out1\"],\"side\":\"RIGHT\"},\"type\":\"ConnectorPlacement.EquallySpacedRectSide\",\"uuid\":\"bbe755dc-37e6-4ccf-babc-f69c624e3127\"},{\"content\":{\"side\":\"TOP\"},\"type\":\"ConnectorPlacement.EquallySpacedRectSide\",\"uuid\":\"af29013d-bc34-4ea7-a3b1-8488eaa61b9f\"}]},\"type\":\"ConnectorPlacement.EquallySpacedConnector\",\"uuid\":\"0c1b5d18-eb5c-4f03-ad77-d46c7555bc12\"}],\"packageUris\":[\"http://schema.mathworks.com/mf0/Connector/R2020b\"],\"version\":\"1.0\"}"
  localization : Subsystem  mask{ekfRate=50}
      settings: PortSchema="{\"entries\":[{\"content\":{\"headerSize\":26,\"margin\":15,\"minimumSpacing\":25,\"sides\":[{\"content\":{\"connectorIds\":[\"In1\",\"In2\",\"In3\"]},\"type\":\"ConnectorPlacement.EquallySpacedRectSide\",\"uuid\":\"200c6e72-70f4-4dab-9973-1633f40310af\"},{\"content\":{\"connectorIds\":[\"Out1\"],\"side\":\"RIGHT\"},\"type\":\"ConnectorPlacement.EquallySpacedRectSide\",\"uuid\":\"bbe755dc-37e6-4ccf-babc-f69c624e3127\"},{\"content\":{\"side\":\"TOP\"},\"type\":\"ConnectorPlacement.EquallySpacedRectSide\",\"uuid\":\"af29013d-bc34-4ea7-a3b1-8488eaa61b9f\"}]},\"type\":\"ConnectorPlacement.EquallySpacedConnector\",\"uuid\":\"0c1b5d18-eb5c-4f03-ad77-d46c7555bc12\"}],\"packageUris\":[\"http://schema.mathworks.com/mf0/Connector/R2020b\"],\"version\":\"1.0\"}"
  safetyManager : Subsystem  mask{batteryEstopTemperature=323.15, batteryShutdownTemperature=333.15}
      settings: PortSchema="{\"entries\":[{\"content\":{\"headerSize\":26,\"margin\":15,\"minimumSpacing\":25,\"sides\":[{\"content\":{\"connectorIds\":[\"In1\"]},\"type\":\"ConnectorPlacement.EquallySpacedRectSide\",\"uuid\":\"200c6e72-70f4-4dab-9973-1633f40310af\"},{\"content\":{\"connectorIds\":[\"Out1\"],\"side\":\"RIGHT\"},\"type\":\"ConnectorPlacement.EquallySpacedRectSide\",\"uuid\":\"bbe755dc-37e6-4ccf-babc-f69c624e3127\"},{\"content\":{\"side\":\"TOP\"},\"type\":\"ConnectorPlacement.EquallySpacedRectSide\",\"uuid\":\"af29013d-bc34-4ea7-a3b1-8488eaa61b9f\"}]},\"type\":\"ConnectorPlacement.EquallySpacedConnector\",\"uuid\":\"0c1b5d18-eb5c-4f03-ad77-d46c7555bc12\"}],\"packageUris\":[\"http://schema.mathworks.com/mf0/Connector/R2020b\"],\"version\":\"1.0\"}"
  twistMux : Subsystem  mask{inputTimeout=0.5}
      settings: PortSchema="{\"entries\":[{\"content\":{\"headerSize\":26,\"margin\":15,\"minimumSpacing\":25,\"sides\":[{\"content\":{\"connectorIds\":[\"In1\",\"In2\",\"In3\"]},\"type\":\"ConnectorPlacement.EquallySpacedRectSide\",\"uuid\":\"200c6e72-70f4-4dab-9973-1633f40310af\"},{\"content\":{\"connectorIds\":[\"Out1\"],\"side\":\"RIGHT\"},\"type\":\"ConnectorPlacement.EquallySpacedRectSide\",\"uuid\":\"bbe755dc-37e6-4ccf-babc-f69c624e3127\"},{\"content\":{\"side\":\"TOP\"},\"type\":\"ConnectorPlacement.EquallySpacedRectSide\",\"uuid\":\"af29013d-bc34-4ea7-a3b1-8488eaa61b9f\"}]},\"type\":\"ConnectorPlacement.EquallySpacedConnector\",\"uuid\":\"0c1b5d18-eb5c-4f03-ad77-d46c7555bc12\"}],\"packageUris\":[\"http://schema.mathworks.com/mf0/Connector/R2020b\"],\"version\":\"1.0\"}"
  Bus Element Out1 : Outport  PortName=localization_odomOut
  Bus Element Out2 : Outport  Port=2  PortName=batteryMonitor_statusOut
  wires:
  Bus Element In1/1 -> twistMux/1(webIn)
  crsfTeleop/1(cmdOut) -> twistMux/2(rcIn)
  Bus Element In2/1 -> twistMux/3(navIn)
  twistMux/1(cmdOut) -> driveController/1(cmdIn)
  driveController/1(odomOut) -> localization/1(wheelOdomIn)
  Bus Element In3/1 -> localization/2(imuIn)
  Bus Element In4/1 -> localization/3(fixIn)
  localization/1(odomOut) -> Bus Element Out1/1
  Bus Element In5/1 -> crsfTeleop/1(crsfIn)
  Bus Element In6/1 -> batteryMonitor/1(bmsIn)
  batteryMonitor/1(statusOut) -> safetyManager/1(batteryIn), Bus Element Out2/1

== system RoverA1Arch/rc ==
  Bus Element Out1 : Outport  PortName=crsfOut

== system RoverA1Arch/safetyController ==
  Bus Element In1 : Inport  PortName=modbus

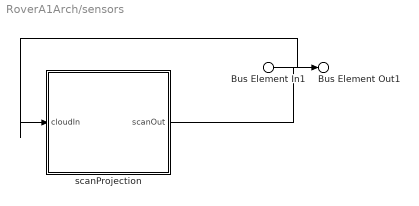
== system RoverA1Arch/sensors ==
  Bus Element In1 : Inport  PortName=scanProjection_cloudIn
  scanProjection : Subsystem
      settings: PortSchema="{\"entries\":[{\"content\":{\"headerSize\":26,\"margin\":15,\"minimumSpacing\":25,\"sides\":[{\"content\":{\"connectorIds\":[\"In1\"]},\"type\":\"ConnectorPlacement.EquallySpacedRectSide\",\"uuid\":\"200c6e72-70f4-4dab-9973-1633f40310af\"},{\"content\":{\"connectorIds\":[\"Out1\"],\"side\":\"RIGHT\"},\"type\":\"ConnectorPlacement.EquallySpacedRectSide\",\"uuid\":\"bbe755dc-37e6-4ccf-babc-f69c624e3127\"},{\"content\":{\"side\":\"TOP\"},\"type\":\"ConnectorPlacement.EquallySpacedRectSide\",\"uuid\":\"af29013d-bc34-4ea7-a3b1-8488eaa61b9f\"}]},\"type\":\"ConnectorPlacement.EquallySpacedConnector\",\"uuid\":\"0c1b5d18-eb5c-4f03-ad77-d46c7555bc12\"}],\"packageUris\":[\"http://schema.mathworks.com/mf0/Connector/R2020b\"],\"version\":\"1.0\"}"
  Bus Element Out1 : Outport  PortName=scanProjection_scanOut
  wires:
  Bus Element In1/1 -> scanProjection/1(cloudIn)
  scanProjection/1(scanOut) -> Bus Element Out1/1

== system RoverA1Arch/driveInterface/driveUi ==
  Bus Element In1 : Inport  PortName=batteryIn
  Bus Element Out1 : Outport  PortName=cmdOut

== system RoverA1Arch/drive_1/controller ==
  Bus Element In1 : Inport  PortName=wheelCmdIn
  Bus Element In2 : Inport  Port=2  PortName=powerIn

== system RoverA1Arch/drive_1/motor ==

== system RoverA1Arch/drive_1/wheel ==

== system RoverA1Arch/drive_2/controller ==
  Bus Element In1 : Inport  PortName=wheelCmdIn
  Bus Element In2 : Inport  Port=2  PortName=powerIn

== system RoverA1Arch/drive_2/motor ==

== system RoverA1Arch/drive_2/wheel ==

== system RoverA1Arch/drive_3/controller ==
  Bus Element In1 : Inport  PortName=wheelCmdIn
  Bus Element In2 : Inport  Port=2  PortName=powerIn

== system RoverA1Arch/drive_3/motor ==

== system RoverA1Arch/drive_3/wheel ==

== system RoverA1Arch/drive_4/controller ==
  Bus Element In1 : Inport  PortName=wheelCmdIn
  Bus Element In2 : Inport  Port=2  PortName=powerIn

== system RoverA1Arch/drive_4/motor ==

== system RoverA1Arch/drive_4/wheel ==

== system RoverA1Arch/orchestrator/navigation ==
  Bus Element In1 : Inport  PortName=odomIn
  Bus Element In2 : Inport  Port=2  PortName=scanIn
  Bus Element Out1 : Outport  PortName=cmdOut

== system RoverA1Arch/platform/batteryMonitor ==
  Bus Element In1 : Inport  PortName=bmsIn
  Bus Element Out1 : Outport  PortName=statusOut

== system RoverA1Arch/platform/crsfTeleop ==
  Bus Element In1 : Inport  PortName=crsfIn
  Bus Element Out1 : Outport  PortName=cmdOut

== system RoverA1Arch/platform/driveController ==
  Bus Element In1 : Inport  PortName=cmdIn
  Bus Element Out1 : Outport  PortName=odomOut

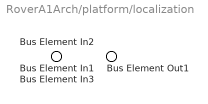
== system RoverA1Arch/platform/localization ==
  Bus Element In1 : Inport  PortName=wheelOdomIn
  Bus Element In2 : Inport  Port=2  PortName=imuIn
  Bus Element In3 : Inport  Port=3  PortName=fixIn
  Bus Element Out1 : Outport  PortName=odomOut

== system RoverA1Arch/platform/safetyManager ==
  Bus Element In1 : Inport  PortName=batteryIn
  Bus Element Out1 : Outport  PortName=modbus

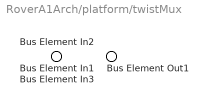
== system RoverA1Arch/platform/twistMux ==
  Bus Element In1 : Inport  PortName=webIn
  Bus Element In2 : Inport  Port=2  PortName=rcIn
  Bus Element In3 : Inport  Port=3  PortName=navIn
  Bus Element Out1 : Outport  PortName=cmdOut

== system RoverA1Arch/sensors/scanProjection ==
  Bus Element In1 : Inport  PortName=cloudIn
  Bus Element Out1 : Outport  PortName=scanOut
